simulink model "Questao_2_Bacterias"  (R2022a)
settings: Solver=VariableStepAuto  StartTime=0.0  StopTime=1  RelTol=1e-3
settings Model: Creator=luanv  LastModifiedBy=luanv

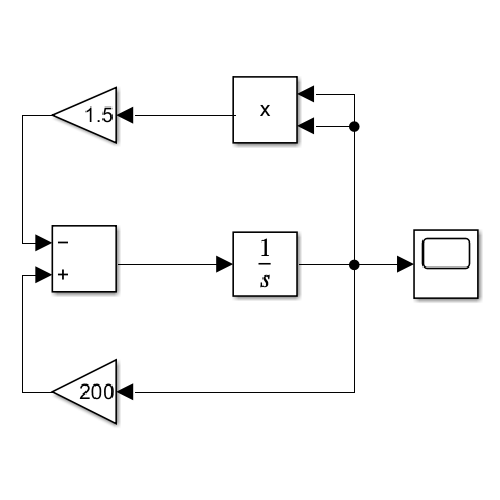
[thumbnail: Simulink's stored preview of the top-level diagram]
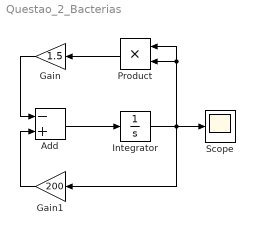
== system Questao_2_Bacterias ==
  Add : Sum  Inputs=-+
  Gain : Gain  Gain=1.5
  Gain1 : Gain  Gain=200
  Integrator : Integrator  InitialCondition=100
  Product : Product
  Scope : Scope
  wires:
  Add/1 -> Integrator/1
  Integrator/1 -> Scope/1, Gain1/1, Product/1, Product/2
  Product/1 -> Gain/1
  Gain1/1 -> Add/2
  Gain/1 -> Add/1
